simulink model "lab1_afak"  (R2021a)
settings: Solver=VariableStepAuto  StartTime=0.0  StopTime=30  MaxStep=0.001  RelTol=1e-3
settings Model: Creator=afayeed  LastModifiedBy=afayeed

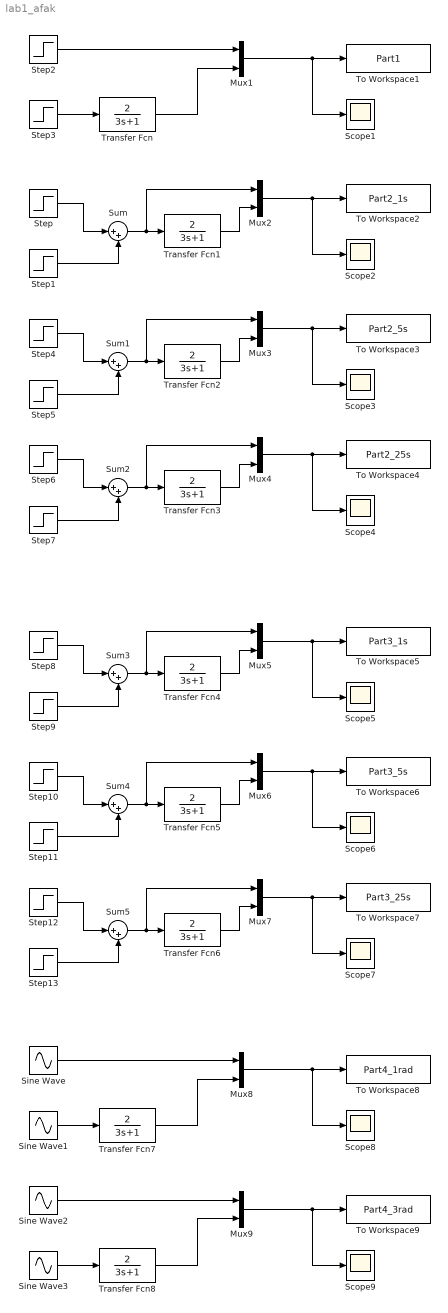
== system lab1_afak ==
  Mux{1..9} (9 alike) : Mux  Inputs=2
  Scope{1..9} (9 alike) : Scope
  Sine Wave : Sin  Bias=2  SampleTime=0
  Sine Wave1 : Sin  Bias=2  SampleTime=0
  Sine Wave2 : Sin  Bias=2  Frequency=3  SampleTime=0
  Sine Wave3 : Sin  Bias=2  Frequency=3  SampleTime=0
  Step{,2..4,6,8,10,12} (8 alike) : Step  Time=3  After=3  SampleTime=0
  Step1 : Step  Time=4  After=-3  SampleTime=0
  Step11 : Step  Time=8  After=3  SampleTime=0
  Step13 : Step  Time=28  After=3  SampleTime=0
  Step5 : Step  Time=8  After=-3  SampleTime=0
  Step7 : Step  Time=28  After=-3  SampleTime=0
  Step9 : Step  Time=4  After=3  SampleTime=0
  Sum{,1..5} (6 alike) : Sum  Inputs=|++
  To Workspace1 : ToWorkspace  VariableName=Part1  SampleTime=-1
  To Workspace2 : ToWorkspace  VariableName=Part2_1s  SampleTime=-1
  To Workspace3 : ToWorkspace  VariableName=Part2_5s  SampleTime=-1
  To Workspace4 : ToWorkspace  VariableName=Part2_25s  SampleTime=-1
  To Workspace5 : ToWorkspace  VariableName=Part3_1s  SampleTime=-1
  To Workspace6 : ToWorkspace  VariableName=Part3_5s  SampleTime=-1
  To Workspace7 : ToWorkspace  VariableName=Part3_25s  SampleTime=-1
  To Workspace8 : ToWorkspace  VariableName=Part4_1rad  SampleTime=-1
  To Workspace9 : ToWorkspace  VariableName=Part4_3rad  SampleTime=-1
  Transfer Fcn{,1..8} (9 alike) : TransferFcn  Numerator=2  Denominator=[3 1]
  wires:
  Step2/1 -> Mux1/1
  Step3/1 -> Transfer Fcn/1
  Transfer Fcn/1 -> Mux1/2
  Mux1/1 -> Scope1/1, To Workspace1/1
  Step/1 -> Sum/1
  Step1/1 -> Sum/2
  Sum/1 -> Transfer Fcn1/1, Mux2/1
  Transfer Fcn1/1 -> Mux2/2
  Mux2/1 -> Scope2/1, To Workspace2/1
  Step5/1 -> Sum1/2
  Sum1/1 -> Transfer Fcn2/1, Mux3/1
  Step4/1 -> Sum1/1
  Mux3/1 -> Scope3/1, To Workspace3/1
  Transfer Fcn2/1 -> Mux3/2
  Mux4/1 -> Scope4/1, To Workspace4/1
  Step6/1 -> Sum2/1
  Step7/1 -> Sum2/2
  Sum2/1 -> Transfer Fcn3/1, Mux4/1
  Transfer Fcn3/1 -> Mux4/2
  Step9/1 -> Sum3/2
  Transfer Fcn6/1 -> Mux7/2
  Sum5/1 -> Transfer Fcn6/1, Mux7/1
  Step13/1 -> Sum5/2
  Step12/1 -> Sum5/1
  Mux7/1 -> Scope7/1, To Workspace7/1
  Sum3/1 -> Transfer Fcn4/1, Mux5/1
  Mux6/1 -> Scope6/1, To Workspace6/1
  Step10/1 -> Sum4/1
  Step11/1 -> Sum4/2
  Sum4/1 -> Transfer Fcn5/1, Mux6/1
  Transfer Fcn5/1 -> Mux6/2
  Step8/1 -> Sum3/1
  Mux5/1 -> Scope5/1, To Workspace5/1
  Transfer Fcn4/1 -> Mux5/2
  Transfer Fcn7/1 -> Mux8/2
  Sine Wave/1 -> Mux8/1
  Mux8/1 -> Scope8/1, To Workspace8/1
  Sine Wave1/1 -> Transfer Fcn7/1
  Mux9/1 -> Scope9/1, To Workspace9/1
  Transfer Fcn8/1 -> Mux9/2
  Sine Wave3/1 -> Transfer Fcn8/1
  Sine Wave2/1 -> Mux9/1
